simulink model "model_dyskretny_1_for_print"  (R2020a)
settings: Solver=VariableStepAuto  StartTime=0.0  StopTime=10.0  RelTol=1e-3
values from neighbouring files (symbols this model uses):
  T = 0.5    [pom.m]    (also in zad1_10.m; zad1_4.m; zad1_6_1.m; zad1_6_2.m)
settings Model: Creator=jakub  LastModifiedBy=jakub

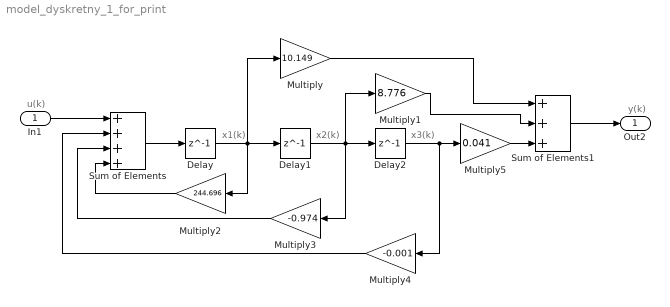
== system model_dyskretny_1_for_print ==
  note: x1(k)
  note: u(k)
  note: x2(k)
  note: x3(k)
  note: y(k)
  In1 : Inport
  Delay : Delay  DelayLength=1  InitialCondition=0  SampleTime=T
  Delay1 : Delay  DelayLength=1  InitialCondition=0  SampleTime=T
  Delay2 : Delay  DelayLength=1  InitialCondition=0  SampleTime=T
  Multiply : Gain  Gain=10.149
  Multiply1 : Gain  Gain=8.776
  Multiply2 : Gain  Gain=244.696
  Multiply3 : Gain  Gain=-0.974
  Multiply4 : Gain  Gain=-0.001
  Multiply5 : Gain  Gain=0.041
  Sum of Elements : Sum  Inputs=++++
  Sum of Elements1 : Sum  Inputs=+++
  Out2 : Outport
  wires:
  In1/1 -> Sum of Elements/1
  Delay/1 -> Multiply2/1, Multiply/1, Delay1/1
  Sum of Elements/1 -> Delay/1
  Delay1/1 -> Multiply1/1, Multiply3/1, Delay2/1
  Delay2/1 -> Multiply4/1, Multiply5/1
  Multiply2/1 -> Sum of Elements/4
  Multiply5/1 -> Sum of Elements1/3
  Multiply3/1 -> Sum of Elements/3
  Multiply4/1 -> Sum of Elements/2
  Multiply1/1 -> Sum of Elements1/2
  Multiply/1 -> Sum of Elements1/1
  Sum of Elements1/1 -> Out2/1
